simulink model "sim_4_twolink_impedance_control"  (R2021a)
settings: Solver=VariableStepAuto  StartTime=0.0  StopTime=12  MaxStep=0.01  RelTol=1e-3
values from neighbouring files (symbols this model uses):
  b1 = 0.01    [sim_params.m]    (also in sim_params_force.m)
  b2 = 0.01    [sim_params.m]    (also in sim_params_force.m)
  D = [zeros(n); eye(n)]    [control_comparison_script.m]    (also in gen_twolink_ss.m = reshape([0.0,0.0,0.0,0.0,0.0,0.0,0.0,0.0],[4,2]))
  g = 9.80665    [sim_params.m]    (also in sim_params_force.m)
  L1x = 0.3    [sim_params.m]    (also in sim_params_force.m)
  L1y = 0.050    (= 0.05)    [sim_params.m]    (also in sim_params_force.m)
  L1z = 0.05    [sim_params.m]    (also in sim_params_force.m)
  L2x = 0.15    [sim_params.m]    (also in sim_params_force.m = 0.3)
  L2y = 0.05    [sim_params.m]    (also in sim_params_force.m)
  L2z = 0.05    [sim_params.m]    (also in sim_params_force.m)
  m1 = m1*1.25    [control_comparison_script.m]    (also in sim_params.m = 2.775; sim_params_force.m = 2.775)
  m2 = m2*1.25    [control_comparison_script.m]    (also in sim_params.m = 1.3875; sim_params_force.m = 2.775)
  max_joint_torque1 = 20    [sim_params.m]    (also in sim_params_force.m)
  max_joint_torque2 = 10    [sim_params.m]    (also in sim_params_force.m = 20)
  theta1_0 = 0    [sim_params.m]    (also in sim_params_force.m = 1.57079632679)
  theta1_dot_0 = 0    [sim_params.m]    (also in sim_params_force.m)
  theta2_0 = 0    [sim_params.m]    (also in sim_params_force.m = -1.57079632679)
  theta2_dot_0 = 0    [sim_params.m]    (also in sim_params_force.m)
undefined symbols (not defined in the file or in its folder): FT_control, Impedance_no, Kdt, Ke_d, Ke_s, Kpt, Levenberg, Marquardt, Mt_inv, R_env, sigbuilder_block, W_env, X, Xenv, Y, Z
libraries: sm_lib x77, nesl_utility x58, pid_lib x6, simulink x6, robotmaniplib x3, robotcorelib x1
(part 5 of 5)

== system sim_4_twolink_impedance_control/Robot+Environment/ARM+curve Simscape/Saturate Inputs ==
  inp : Inport
  Demux : Demux  Outputs=2
  Mux : Mux  Inputs=2
  Saturate Gripper Force : Saturate  UpperLimit=max_joint_torque2  LowerLimit=-max_joint_torque2
  Saturate Joint Torques : Saturate  UpperLimit=max_joint_torque1  LowerLimit=-max_joint_torque1
  sat : Outport  VectorParamsAs1DForOutWhenUnconnected=off
  wires:
  Saturate Joint Torques/1 -> Mux/1
  Demux/1 -> Saturate Joint Torques/1
  Mux/1 -> sat/1
  Saturate Gripper Force/1 -> Mux/2
  inp/1 -> Demux/1
  Demux/2 -> Saturate Gripper Force/1

== system sim_4_twolink_impedance_control/Robot+Environment/ARM+extrude Simscape/Saturate Inputs ==
  inp : Inport
  Demux : Demux  Outputs=2
  Mux : Mux  Inputs=2
  Saturate Gripper Force : Saturate  UpperLimit=max_joint_torque2  LowerLimit=-max_joint_torque2
  Saturate Joint Torques : Saturate  UpperLimit=max_joint_torque1  LowerLimit=-max_joint_torque1
  sat : Outport  VectorParamsAs1DForOutWhenUnconnected=off
  wires:
  Saturate Joint Torques/1 -> Mux/1
  Demux/1 -> Saturate Joint Torques/1
  Mux/1 -> sat/1
  Saturate Gripper Force/1 -> Mux/2
  inp/1 -> Demux/1
  Demux/2 -> Saturate Gripper Force/1

== system sim_4_twolink_impedance_control/Robot+Environment/ARM+no constraints Simscape/Saturate Inputs ==
  inp : Inport
  Demux : Demux  Outputs=2
  Mux : Mux  Inputs=2
  Saturate Gripper Force : Saturate  UpperLimit=max_joint_torque2  LowerLimit=-max_joint_torque2
  Saturate Joint Torques : Saturate  UpperLimit=max_joint_torque1  LowerLimit=-max_joint_torque1
  sat : Outport  VectorParamsAs1DForOutWhenUnconnected=off
  wires:
  Saturate Joint Torques/1 -> Mux/1
  Demux/1 -> Saturate Joint Torques/1
  Mux/1 -> sat/1
  Saturate Gripper Force/1 -> Mux/2
  inp/1 -> Demux/1
  Demux/2 -> Saturate Gripper Force/1

== system sim_4_twolink_impedance_control/Robot+Environment/ARM+ramp up Simscape/Saturate Inputs ==
  inp : Inport
  Demux : Demux  Outputs=2
  Mux : Mux  Inputs=2
  Saturate Gripper Force : Saturate  UpperLimit=max_joint_torque2  LowerLimit=-max_joint_torque2
  Saturate Joint Torques : Saturate  UpperLimit=max_joint_torque1  LowerLimit=-max_joint_torque1
  sat : Outport  VectorParamsAs1DForOutWhenUnconnected=off
  wires:
  Saturate Joint Torques/1 -> Mux/1
  Demux/1 -> Saturate Joint Torques/1
  Mux/1 -> sat/1
  Saturate Gripper Force/1 -> Mux/2
  inp/1 -> Demux/1
  Demux/2 -> Saturate Gripper Force/1

== system sim_4_twolink_impedance_control/Trajectory/Step command/Joint commands ==
  Demux : Demux  Tag=STV Demux  Outputs=2
      settings: DisplayOption=none
  FromWs : FromWorkspace  Tag=STV FromWs  VariableName=tuvar
      SigBuilderData=|
      | common.afterFinalStr = 'Extrapolate'
      | common.sampleTime = 0
      | dataSet(1).timeRange = [0 1000]
      | dataSet(1).name = 'PULSES_SMALL'
      | dataSet(2).timeRange = [0 1000]
      | dataSet(2).name = 'ZERO'
      | dataSet(3).timeRange = [0 1000]
      | dataSet(3).name = 'PULSES_BIG'
      | dataSet(4).timeRange = [0 1000]
      | dataSet(4).name = 'PULSES_SMALL1'
      | sbobj.Groups(1).Name = 'PULSES_SMALL'
      | sbobj.Groups(1).Signals(1).Name = 'cmd_x'
      | sbobj.Groups(1).Signals(1).XData = [0 2.4 2.4 5.05 8.1 8.1 1000]
      | sbobj.Groups(1).Signals(1).YData = [0.2 0.2 0.299 0.299 0.299 0.2 0.2]
      | sbobj.Groups(1).Signals(2).Name = 'cmd_y'
      | sbobj.Groups(1).Signals(2).XData = [0 2.4 2.4 5.05 8.1 8.1 1000]
      | sbobj.Groups(1).Signals(2).YData = [0.2 0.2 0.299 0.299 0.299 0.2 0.2]
      | sbobj.Groups(1).TimeRange = [0 1000]
      | sbobj.Groups(2).Name = 'ZERO'
      | sbobj.Groups(2).Signals(1).Name = 'cmd_x'
      | sbobj.Groups(2).Signals(1).XData = [0 500 500 1000]
      | sbobj.Groups(2).Signals(1).YData = [0 0 1 1]
      | sbobj.Groups(2).Signals(2).Name = 'cmd_y'
      | sbobj.Groups(2).Signals(2).XData = [0 1000]
      | sbobj.Groups(2).Signals(2).YData = [0 0]
      | sbobj.Groups(2).TimeRange = [0 1000]
      | sbobj.Groups(3).Name = 'PULSES_BIG'
      | sbobj.Groups(3).Signals(1).Name = 'cmd_x'
      | sbobj.Groups(3).Signals(1).XData = [0 500 500 1000]
      | sbobj.Groups(3).Signals(1).YData = [0 0 1 1]
      | sbobj.Groups(3).Signals(2).Name = 'cmd_y'
      | sbobj.Groups(3).Signals(2).XData = [0 1000]
      | sbobj.Groups(3).Signals(2).YData = [0 0]
      | sbobj.Groups(3).TimeRange = [0 1000]
      | sbobj.Groups(4).Name = 'PULSES_SMALL1'
      | sbobj.Groups(4).Signals(1).Name = 'cmd_x'
      | sbobj.Groups(4).Signals(1).XData = [0 500 500 1000]
      | sbobj.Groups(4).Signals(1).YData = [0 0 1 1]
      | sbobj.Groups(4).Signals(2).Name = 'cmd_y'
      | sbobj.Groups(4).Signals(2).XData = [0 1000]
      | sbobj.Groups(4).Signals(2).YData = [0 0]
      | sbobj.Groups(4).TimeRange = [0 1000]
  cmd_x : Outport  Tag=STV Outport
  cmd_y : Outport  Tag=STV Outport  Port=2
  wires:
  FromWs/1 -> Demux/1
  Demux/1 -> cmd_x/1
  Demux/2 -> cmd_y/1

== matlab function sim_4_twolink_impedance_control/Forward Kinmatics/Jacobian1 ==
  data: L_1 input; J output; L_2 input; theta_1 input; theta_2 input
function J = jacobian_geom(L_1,L_2,theta_1,theta_2)

J = [
       -L_1.*sin(theta_1)-L_2.*sin(theta_1+theta_2) , -L_2.*sin(theta_1+theta_2) ;
        L_1.*cos(theta_1)+L_2.*cos(theta_1+theta_2) ,  L_2.*cos(theta_1+theta_2) ;
    ];

== matlab function sim_4_twolink_impedance_control/Robot+Environment/ARM+Wall Simulink/Jacobian1 ==
  data: L_1 input; J output; L_2 input; theta_1 input; theta_2 input
function J = jacobian_geom(L_1,L_2,theta_1,theta_2)

J = [
       -L_1.*sin(theta_1)-L_2.*sin(theta_1+theta_2) , -L_2.*sin(theta_1+theta_2) ;
        L_1.*cos(theta_1)+L_2.*cos(theta_1+theta_2) ,  L_2.*cos(theta_1+theta_2) ;
    ];

== matlab function sim_4_twolink_impedance_control/Robot+Environment/ARM+Wall Simulink/MATLAB Function ==
  data: x input; F output; xe input; x_dot input; Ks input; Kd input; y input; W_env input
function F = env_force(x,xe,x_dot,Ks,Kd,y,W_env)
% environment modeled as spring with stiffness Ks and damping Kd
% if no contact, no exerted force
% env is a wall of width W_env
F=0;
if (x-xe)>0 && abs(y)<(W_env/2)
    F= Ks*(x-xe)+Kd*(x_dot-0);
end

== matlab function sim_4_twolink_impedance_control/Inverse Kinmatics/IK/Inverse Kinematics ==
  data: x input; q1 output; y input; L1 input; L2 input; q2 output
function [q1, q2]= ik_rr(x,y,L1,L2)
%IK_RR 


tmp = (x^2+y^2-L1^2-L2^2)/(2*L1*L2);
if abs(tmp-1)<0.0001
    tmp = 1;
end

if abs(tmp)>1
    q2=0;
else
    q2 = acos(tmp);
    if isnan(q2) || isinf(q2) || ~isreal(q2)
        q2 = 0;
    end
end

q1 = atan2(y,x)-atan2(L2*sin(q2), L1+L2*cos(q2));
if isnan(q1) || isinf(q1) || ~isreal(q1)
    q1 = 0;
end

== matlab function sim_4_twolink_impedance_control/Robot+Environment/ARM+Wall Simulink/Forward Kinematics ==
  data: L_1 input; XE output; L_2 input; theta_1 input; theta_2 input; YE output
function [XE,YE] = FK(L_1,L_2,theta_1,theta_2)

XE = L_2.*cos(theta_1+theta_2)+L_1.*cos(theta_1);
if nargout > 1
    YE = L_2.*sin(theta_1+theta_2)+L_1.*sin(theta_1);
end

== matlab function sim_4_twolink_impedance_control/Forward Kinmatics/Forward Kinematics ==
  data: L_1 input; XE output; L_2 input; theta_1 input; theta_2 input; YE output
function [XE,YE] = FK(L_1,L_2,theta_1,theta_2)

XE = L_2.*cos(theta_1+theta_2)+L_1.*cos(theta_1);
if nargout > 1
    YE = L_2.*sin(theta_1+theta_2)+L_1.*sin(theta_1);
end

== matlab function sim_4_twolink_impedance_control/Controller/Impedance (with F//T) +Inverse Dynamics control /Jacobian dot/ Jacobian dot ==
  data: L_1 input; J_dot output; L_2 input; th1 input; th2 input; th1_d input; th2_d input
function J_dot = jacobian_dot(L_1,L_2,th1,th2,th1_d, th2_d)

J_dot = [
    [- L_2*cos(th1 + th2)*(th1_d + th2_d) - L_1*th1_d*cos(th1), -L_2*cos(th1 + th2)*(th1_d + th2_d)];
    [- L_1*th1_d*sin(th1) - L_2*sin(th1 + th2)*(th1_d + th2_d), -L_2*sin(th1 + th2)*(th1_d + th2_d)];
];

== matlab function sim_4_twolink_impedance_control/Controller/Simple complaince Control/MCKGQ ==
  data: L_1x input; M output; L_1y input; L_2x input; L_2y input; b1 input; b2 input; g input; m1 input; m2 input; q1 input; q2 input; q1_D input; q2_D input; tau1 input; tau2 input; C output; K output; G output; Q output
function [M,C,K,G,Q] = MCKGQ(L_1x,L_1y,L_2x,L_2y,b1,b2,g,m1,m2,q1,q2,q1_D,q2_D,tau1,tau2)
%#codegen

%    This function was generated by the Symbolic Math Toolbox version 8.7.
%    30-May-2022 13:59:37

M = reshape([(L_1x.^2.*m1)./3.0+L_1x.^2.*m2+(L_1y.^2.*m1)./1.2e+1+(L_2x.^2.*m2)./4.0+L_1x.*L_2x.*m2.*cos(q2),(L_2x.*m2.*(L_2x+L_1x.*cos(q2).*2.0))./4.0,(L_2x.*m2.*(L_2x+L_1x.*cos(q2).*2.0))./4.0,(m2.*(L_2x.^2.*4.0+L_2y.^2))./1.2e+1],[2,2]);
if nargout > 1
    C = reshape([-L_1x.*L_2x.*m2.*q2_D.*sin(q2),(L_1x.*L_2x.*m2.*q1_D.*sin(q2))./2.0,L_1x.*L_2x.*m2.*q2_D.*sin(q2).*(-1.0./2.0),0.0],[2,2]);
end
if nargout > 2
    K = reshape([0.0,0.0,0.0,0.0],[2,2]);
end
if nargout > 3
    G = [(g.*(L_2x.*m2.*cos(q1+q2)+L_1x.*m1.*cos(q1)+L_1x.*m2.*cos(q1).*2.0))./2.0;(L_2x.*g.*m2.*cos(q1+q2))./2.0];
end
if nargout > 4
    Q = [tau1-b1.*q1_D;tau2-b2.*q2_D];
end

== matlab function sim_4_twolink_impedance_control/Controller/Impedance (with F//T) +Inverse Dynamics control /inverse jacobian1/Inverse Jacobian ==
  data: L_1 input; inv_J output; L_2 input; th1 input; th2 input
function inv_J = inv_jacobian(L_1,L_2,th1,th2)

inv_J = [
% [                            -cos(th1 + th2)/(L_1*cos(th1 + th2)*sin(th1) - L_1*sin(th1 + th2)*cos(th1)),                             -sin(th1 + th2)/(L_1*cos(th1 + th2)*sin(th1) - L_1*sin(th1 + th2)*cos(th1))];
% [(L_2*cos(th1 + th2) + L_1*cos(th1))/(L_1*L_2*cos(th1 + th2)*sin(th1) - L_1*L_2*sin(th1 + th2)*cos(th1)), (L_2*sin(th1 + th2) + L_1*sin(th1))/(L_1*L_2*cos(th1 + th2)*sin(th1) - L_1*L_2*sin(th1 + th2)*cos(th1))];
[                          cos(th1 + th2)/(L_1*sin(th2)),                           sin(th1 + th2)/(L_1*sin(th2))];
[-(L_2*cos(th1 + th2) + L_1*cos(th1))/(L_1*L_2*sin(th2)), -(L_2*sin(th1 + th2) + L_1*sin(th1))/(L_1*L_2*sin(th2))];
];

== matlab function sim_4_twolink_impedance_control/Controller/Impedance (without F//T) + Inverse Dynamics control /Jacobian dot/ Jacobian dot ==
  data: L_1 input; J_dot output; L_2 input; th1 input; th2 input; th1_d input; th2_d input
function J_dot = jacobian_dot(L_1,L_2,th1,th2,th1_d, th2_d)

J_dot = [
    [- L_2*cos(th1 + th2)*(th1_d + th2_d) - L_1*th1_d*cos(th1), -L_2*cos(th1 + th2)*(th1_d + th2_d)];
    [- L_1*th1_d*sin(th1) - L_2*sin(th1 + th2)*(th1_d + th2_d), -L_2*sin(th1 + th2)*(th1_d + th2_d)];
];

== matlab function sim_4_twolink_impedance_control/Controller/Impedance (without F//T) + Inverse Dynamics control /MCKGQ ==
  data: L_1x input; M output; L_1y input; L_2x input; L_2y input; b1 input; b2 input; g input; m1 input; m2 input; q1 input; q2 input; q1_D input; q2_D input; tau1 input; tau2 input; C output; K output; G output; Q output
function [M,C,K,G,Q] = MCKGQ(L_1x,L_1y,L_2x,L_2y,b1,b2,g,m1,m2,q1,q2,q1_D,q2_D,tau1,tau2)
%#codegen

%    This function was generated by the Symbolic Math Toolbox version 8.7.
%    30-May-2022 13:59:37

M = reshape([(L_1x.^2.*m1)./3.0+L_1x.^2.*m2+(L_1y.^2.*m1)./1.2e+1+(L_2x.^2.*m2)./4.0+L_1x.*L_2x.*m2.*cos(q2),(L_2x.*m2.*(L_2x+L_1x.*cos(q2).*2.0))./4.0,(L_2x.*m2.*(L_2x+L_1x.*cos(q2).*2.0))./4.0,(m2.*(L_2x.^2.*4.0+L_2y.^2))./1.2e+1],[2,2]);
if nargout > 1
    C = reshape([-L_1x.*L_2x.*m2.*q2_D.*sin(q2),(L_1x.*L_2x.*m2.*q1_D.*sin(q2))./2.0,L_1x.*L_2x.*m2.*q2_D.*sin(q2).*(-1.0./2.0),0.0],[2,2]);
end
if nargout > 2
    K = reshape([0.0,0.0,0.0,0.0],[2,2]);
end
if nargout > 3
    G = [(g.*(L_2x.*m2.*cos(q1+q2)+L_1x.*m1.*cos(q1)+L_1x.*m2.*cos(q1).*2.0))./2.0;(L_2x.*g.*m2.*cos(q1+q2))./2.0];
end
if nargout > 4
    Q = [tau1-b1.*q1_D;tau2-b2.*q2_D];
end

== matlab function sim_4_twolink_impedance_control/Inverse Kinmatics/Forward Kinmatics/Forward Kinematics ==
  data: L_1 input; XE output; L_2 input; theta_1 input; theta_2 input; YE output
function [XE,YE] = FK(L_1,L_2,theta_1,theta_2)

XE = L_2.*cos(theta_1+theta_2)+L_1.*cos(theta_1);
if nargout > 1
    YE = L_2.*sin(theta_1+theta_2)+L_1.*sin(theta_1);
end

== matlab function sim_4_twolink_impedance_control/Controller/Impedance (without F//T) + Inverse Dynamics control /inverse jacobian1/Inverse Jacobian ==
  data: L_1 input; inv_J output; L_2 input; th1 input; th2 input
function inv_J = inv_jacobian(L_1,L_2,th1,th2)

inv_J = [
% [                            -cos(th1 + th2)/(L_1*cos(th1 + th2)*sin(th1) - L_1*sin(th1 + th2)*cos(th1)),                             -sin(th1 + th2)/(L_1*cos(th1 + th2)*sin(th1) - L_1*sin(th1 + th2)*cos(th1))];
% [(L_2*cos(th1 + th2) + L_1*cos(th1))/(L_1*L_2*cos(th1 + th2)*sin(th1) - L_1*L_2*sin(th1 + th2)*cos(th1)), (L_2*sin(th1 + th2) + L_1*sin(th1))/(L_1*L_2*cos(th1 + th2)*sin(th1) - L_1*L_2*sin(th1 + th2)*cos(th1))];
[                          cos(th1 + th2)/(L_1*sin(th2)),                           sin(th1 + th2)/(L_1*sin(th2))];
[-(L_2*cos(th1 + th2) + L_1*cos(th1))/(L_1*L_2*sin(th2)), -(L_2*sin(th1 + th2) + L_1*sin(th1))/(L_1*L_2*sin(th2))];
];

== matlab function sim_4_twolink_impedance_control/Controller/Impedance (without F//T) + Inverse Dynamics control /Jacobian1/Jacobian ==
  data: L_1 input; J output; L_2 input; theta_1 input; theta_2 input
function J = jacobian_geom(L_1,L_2,theta_1,theta_2)

J = [
       -L_1.*sin(theta_1)-L_2.*sin(theta_1+theta_2) , -L_2.*sin(theta_1+theta_2) ;
        L_1.*cos(theta_1)+L_2.*cos(theta_1+theta_2) ,  L_2.*cos(theta_1+theta_2) ;
    ];

== matlab function sim_4_twolink_impedance_control/Controller/Impedance (with F//T) +Inverse Dynamics control /Jacobian1/Jacobian ==
  data: L_1 input; J output; L_2 input; theta_1 input; theta_2 input
function J = jacobian_geom(L_1,L_2,theta_1,theta_2)

J = [
       -L_1.*sin(theta_1)-L_2.*sin(theta_1+theta_2) , -L_2.*sin(theta_1+theta_2) ;
        L_1.*cos(theta_1)+L_2.*cos(theta_1+theta_2) ,  L_2.*cos(theta_1+theta_2) ;
    ];

== matlab function sim_4_twolink_impedance_control/Robot+Environment/ARM+Wall Simulink/MCKGQ ==
  data: L_1x input; M output; L_1y input; L_2x input; L_2y input; b1 input; b2 input; g input; m1 input; m2 input; q1 input; q2 input; q1_D input; q2_D input; tau1 input; tau2 input; C output; K output; G output; Q output
function [M,C,K,G,Q] = MCKGQ(L_1x,L_1y,L_2x,L_2y,b1,b2,g,m1,m2,q1,q2,q1_D,q2_D,tau1,tau2)
%#codegen

%    This function was generated by the Symbolic Math Toolbox version 8.7.
%    30-May-2022 13:59:37

M = reshape([(L_1x.^2.*m1)./3.0+L_1x.^2.*m2+(L_1y.^2.*m1)./1.2e+1+(L_2x.^2.*m2)./4.0+L_1x.*L_2x.*m2.*cos(q2),(L_2x.*m2.*(L_2x+L_1x.*cos(q2).*2.0))./4.0,(L_2x.*m2.*(L_2x+L_1x.*cos(q2).*2.0))./4.0,(m2.*(L_2x.^2.*4.0+L_2y.^2))./1.2e+1],[2,2]);
if nargout > 1
    C = reshape([-L_1x.*L_2x.*m2.*q2_D.*sin(q2),(L_1x.*L_2x.*m2.*q1_D.*sin(q2))./2.0,L_1x.*L_2x.*m2.*q2_D.*sin(q2).*(-1.0./2.0),0.0],[2,2]);
end
if nargout > 2
    K = reshape([0.0,0.0,0.0,0.0],[2,2]);
end
if nargout > 3
    G = [(g.*(L_2x.*m2.*cos(q1+q2)+L_1x.*m1.*cos(q1)+L_1x.*m2.*cos(q1).*2.0))./2.0;(L_2x.*g.*m2.*cos(q1+q2))./2.0];
end
if nargout > 4
    Q = [tau1-b1.*q1_D;tau2-b2.*q2_D];
end

== matlab function sim_4_twolink_impedance_control/Robot+Environment/ARM+Wall Simulink/MATLAB Function1 ==
  data: M input; the_cond output
function the_cond = COND(M)
%#codegen

the_cond = cond(M);

end

== matlab function sim_4_twolink_impedance_control/Controller/Simple complaince Control/Jacobian1/Jacobian ==
  data: L_1 input; J output; L_2 input; theta_1 input; theta_2 input
function J = jacobian_geom(L_1,L_2,theta_1,theta_2)

J = [
       -L_1.*sin(theta_1)-L_2.*sin(theta_1+theta_2) , -L_2.*sin(theta_1+theta_2) ;
        L_1.*cos(theta_1)+L_2.*cos(theta_1+theta_2) ,  L_2.*cos(theta_1+theta_2) ;
    ];

== matlab function sim_4_twolink_impedance_control/Controller/Impedance (with F//T) +Inverse Dynamics control /MCKGQ ==
  data: L_1x input; M output; L_1y input; L_2x input; L_2y input; b1 input; b2 input; g input; m1 input; m2 input; q1 input; q2 input; q1_D input; q2_D input; tau1 input; tau2 input; C output; K output; G output; Q output
function [M,C,K,G,Q] = MCKGQ(L_1x,L_1y,L_2x,L_2y,b1,b2,g,m1,m2,q1,q2,q1_D,q2_D,tau1,tau2)
%#codegen

%    This function was generated by the Symbolic Math Toolbox version 8.7.
%    30-May-2022 13:59:37

M = reshape([(L_1x.^2.*m1)./3.0+L_1x.^2.*m2+(L_1y.^2.*m1)./1.2e+1+(L_2x.^2.*m2)./4.0+L_1x.*L_2x.*m2.*cos(q2),(L_2x.*m2.*(L_2x+L_1x.*cos(q2).*2.0))./4.0,(L_2x.*m2.*(L_2x+L_1x.*cos(q2).*2.0))./4.0,(m2.*(L_2x.^2.*4.0+L_2y.^2))./1.2e+1],[2,2]);
if nargout > 1
    C = reshape([-L_1x.*L_2x.*m2.*q2_D.*sin(q2),(L_1x.*L_2x.*m2.*q1_D.*sin(q2))./2.0,L_1x.*L_2x.*m2.*q2_D.*sin(q2).*(-1.0./2.0),0.0],[2,2]);
end
if nargout > 2
    K = reshape([0.0,0.0,0.0,0.0],[2,2]);
end
if nargout > 3
    G = [(g.*(L_2x.*m2.*cos(q1+q2)+L_1x.*m1.*cos(q1)+L_1x.*m2.*cos(q1).*2.0))./2.0;(L_2x.*g.*m2.*cos(q1+q2))./2.0];
end
if nargout > 4
    Q = [tau1-b1.*q1_D;tau2-b2.*q2_D];
end
